simulink model "katana_smo"  (R2020a)
settings: Solver=ode8  StartTime=0.0  StopTime=20  FixedStep=0.004  MaxStep=0.004  RelTol=1e-3
InitFcn:
  | [lowpass_B, lowpass_A] = butter(4,1,'s');
  | manipulator_tree = importrobot('../../catkin_ws/src/katana_description/katana_description.urdf');
  | manipulator_tree.Gravity = [0 0 -9.81];
model workspace (MAT data in the model file):
  SL_ROS_VariableLengthArrays_MaxSizes.CommonInfo.ArrayTruncateAction = 'EmitWarning'
  SL_ROS_VariableLengthArrays_MaxSizes.MsgTypeMap = containers.Map
  SL_ROS_VariableLengthArrays_MaxSizes.MsgTypeMap.serialization.keys = {'std_msgs/Float32MultiArray', 'std_msgs/Float64MultiArray'}
  SL_ROS_VariableLengthArrays_MaxSizes.MsgTypeMap.serialization.values{1}.PropertyName = 'Data'
  SL_ROS_VariableLengthArrays_MaxSizes.MsgTypeMap.serialization.values{1}.DataType = 'single'
  SL_ROS_VariableLengthArrays_MaxSizes.MsgTypeMap.serialization.values{1}.MaxLength = 14
  SL_ROS_VariableLengthArrays_MaxSizes.MsgTypeMap.serialization.values{2}.PropertyName = 'Data'
  SL_ROS_VariableLengthArrays_MaxSizes.MsgTypeMap.serialization.values{2}.DataType = 'double'
  SL_ROS_VariableLengthArrays_MaxSizes.MsgTypeMap.serialization.values{2}.MaxLength = 7
  SL_ROS_VariableLengthArrays_MaxSizes.MsgTypeMap.serialization.uniformity = 0
  SL_ROS_VariableLengthArrays_MaxSizes.MsgTypeMap.serialization.keyType = 'char'
  SL_ROS_VariableLengthArrays_MaxSizes.MsgTypeMap.serialization.valueType = 'any'
undefined symbols (not defined in the file or in its folder): Data, Data_SL_Info, lowpass_A, lowpass_B
libraries: robotlib x9, robotmaniplib x3, robotcorelib x1
settings Model: Creator=marco  LastModifiedBy=josea
settings OptimizationCC: EnhancedBackFolding=on  PassReuseOutputArgsAs=Individual arguments  ZeroExternalMemoryAtStartup=off  ZeroInternalMemoryAtStartup=off  MaxStackSize=64  OptimizeBlockOrder=speed  DifferentSizesBufferReuse=on  OptimizationCustomize=off  EfficientTunableParamExpr=on
settings DebuggingCC: ParameterTunabilityLossMsg=error
settings HardwareCC: ProdBitPerLong=64  ProdHWDeviceType=Intel->x86-64 (Linux 64)
settings RTWCC: SystemTargetFile=ert.tlc  HardwareBoard=Robot Operating System (ROS)  TemplateMakefile=ert_default_tmf  Toolchain=Catkin  TargetLang=C++
settings CodeAppCC: ForceParamTrailComments=on  IgnoreCustomStorageClasses=off  OperatorAnnotations=on  SimulinkDataObjDesc=on  SFDataObjDesc=on  InsertBlockDesc=on
settings ERTTargetCC: SupportContinuousTime=on  SupportVariableSizeSignals=on

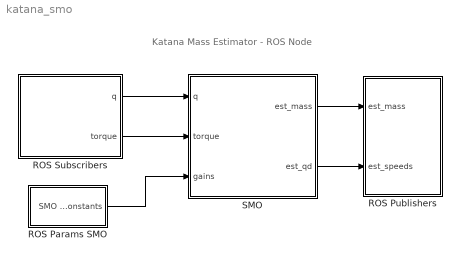
== system katana_smo ==
  note: Katana Mass Estimator - ROS Node
  ROS Params SMO : Subsystem
  ROS Publishers : Subsystem
  ROS Subscribers : Subsystem
  SMO : Subsystem
  wires:
  ROS Subscribers/2(torque) -> SMO/2(torque)
  ROS Subscribers/1(q) -> SMO/1(q)
  ROS Params SMO/1(SMO Constants) -> SMO/3(gains)
  SMO/1(est_mass) -> ROS Publishers/1(est_mass)
  SMO/2(est_qd) -> ROS Publishers/2("est_speeds ")

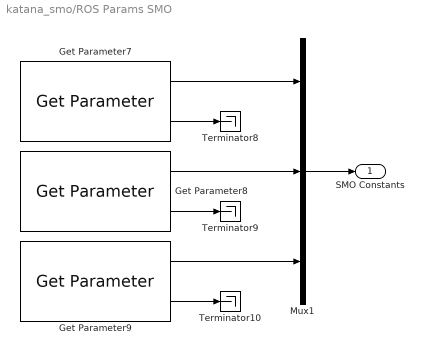
== system katana_smo/ROS Params SMO ==
  Get Parameter7 : robotlib/Get Parameter  ParameterSource=Specify your own  ParameterName=/smo/lambda  ParameterType=double  ParameterMaxArrayLength=16  ParameterInitialValue=0.0  SampleTime=1  ShowErrorCodeOutput=on  ModelName=katana_smo  BlockId=ParamGet_katana_smo_421
      settings: SourceProductBaseCode=RR
  Get Parameter8 : robotlib/Get Parameter  ParameterSource=Specify your own  ParameterName=/smo/alpha  ParameterType=double  ParameterMaxArrayLength=16  ParameterInitialValue=0.0  SampleTime=1  ShowErrorCodeOutput=on  ModelName=katana_smo  BlockId=ParamGet_katana_smo_422
      settings: SourceProductBaseCode=RR
  Get Parameter9 : robotlib/Get Parameter  ParameterSource=Specify your own  ParameterName=/smo/gamma  ParameterType=double  ParameterMaxArrayLength=16  ParameterInitialValue=0.0  SampleTime=1  ShowErrorCodeOutput=on  ModelName=katana_smo  BlockId=ParamGet_katana_smo_423
      settings: SourceProductBaseCode=RR
  Mux1 : Mux  Inputs=3
  Terminator10 : Terminator
  Terminator8 : Terminator
  Terminator9 : Terminator
  SMO Constants : Outport
  wires:
  Get Parameter9/1 -> Mux1/3
  Get Parameter7/1 -> Mux1/1
  Get Parameter7/2 -> Terminator8/1
  Mux1/1 -> SMO Constants/1
  Get Parameter8/2 -> Terminator9/1
  Get Parameter9/2 -> Terminator10/1
  Get Parameter8/1 -> Mux1/2

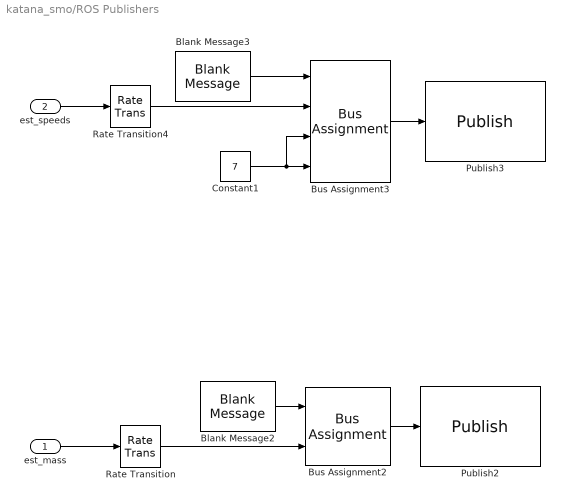
== system katana_smo/ROS Publishers ==
  est_mass : Inport
  "est_speeds " : Inport  Port=2
  Blank Message2 : robotlib/Blank Message  messageClass=Message  entityType=std_msgs/Float64  messageType=std_msgs/Float64  SampleTime=0.04
  Blank Message3 : robotlib/Blank Message  messageClass=Message  entityType=std_msgs/Float64MultiArray  messageType=std_msgs/Float64MultiArray  SampleTime=0.004
  Bus Assignment2 : BusAssignment  AssignedSignals=Data
  Bus Assignment3 : BusAssignment  AssignedSignals=Data,Data_SL_Info.CurrentLength,Data_SL_Info.ReceivedLength
  Constant1 : Constant  Value=7  OutDataTypeStr=uint32  SampleTime=0.004
  Publish2 : robotlib/Publish  topicSource=Specify your own  topic=/estimated_mass  messageType=std_msgs/Float64  messageQueueLength=1
  Publish3 : robotlib/Publish  topicSource=Specify your own  topic=/smo/estimated_speeds  messageType=std_msgs/Float64MultiArray  messageQueueLength=1
  Rate Transition : RateTransition
  Rate Transition4 : RateTransition
  wires:
  Blank Message2/1 -> Bus Assignment2/1
  Rate Transition/1 -> Bus Assignment2/2
  Bus Assignment2/1 -> Publish2/1
  Rate Transition4/1 -> Bus Assignment3/2
  Bus Assignment3/1 -> Publish3/1
  Constant1/1 -> Bus Assignment3/4, Bus Assignment3/3
  Blank Message3/1 -> Bus Assignment3/1
  est_mass/1 -> Rate Transition/1
  "est_speeds "/1 -> Rate Transition4/1

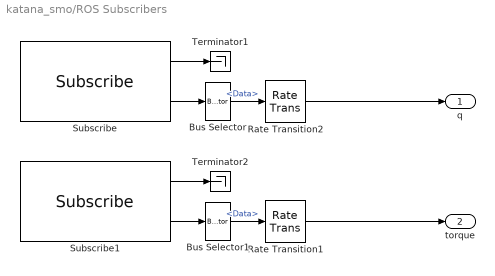
== system katana_smo/ROS Subscribers ==
  Bus Selector : BusSelector  OutputSignals=Data
  Bus Selector1 : BusSelector  OutputSignals=Data
  Rate Transition1 : RateTransition
  Rate Transition2 : RateTransition
  Subscribe : robotlib/Subscribe  topicSource=Specify your own  topic=/joint_positions  messageType=std_msgs/Float64MultiArray  sampleTime=0.004  messageQueueLength=1
  Subscribe1 : robotlib/Subscribe  topicSource=Specify your own  topic=/joint_torques  messageType=std_msgs/Float64MultiArray  sampleTime=0.004  messageQueueLength=1
  Terminator1 : Terminator
  Terminator2 : Terminator
  q : Outport
  torque : Outport  Port=2
  wires:
  Bus Selector/1 -> Rate Transition2/1  "<Data>"
  Rate Transition2/1 -> q/1
  Subscribe/2 -> Bus Selector/1
  Subscribe/1 -> Terminator1/1
  Subscribe1/1 -> Terminator2/1
  Subscribe1/2 -> Bus Selector1/1
  Bus Selector1/1 -> Rate Transition1/1  "<Data>"
  Rate Transition1/1 -> torque/1

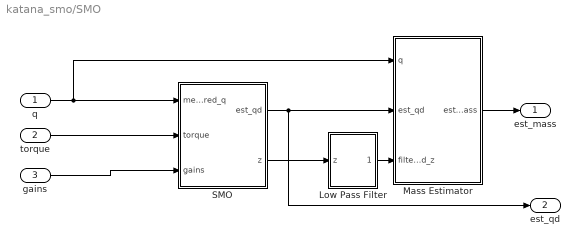
== system katana_smo/SMO ==
  q : Inport
  torque : Inport  Port=2
  gains : Inport  Port=3
  Low Pass Filter : Subsystem
  Mass Estimator : Subsystem
  SMO : Subsystem
  est_mass : Outport
  est_qd : Outport  Port=2
  wires:
  SMO/2(z) -> Low Pass Filter/1(z)
  Mass Estimator/1(est_mass) -> est_mass/1
  torque/1 -> SMO/2(torque)
  q/1 -> Mass Estimator/1(q), SMO/1(measured_q)
  Low Pass Filter/1(filtered) -> Mass Estimator/3(filtered_z)
  gains/1 -> SMO/3(gains)
  SMO/1(est_qd) -> est_qd/1, Mass Estimator/2(est_qd)

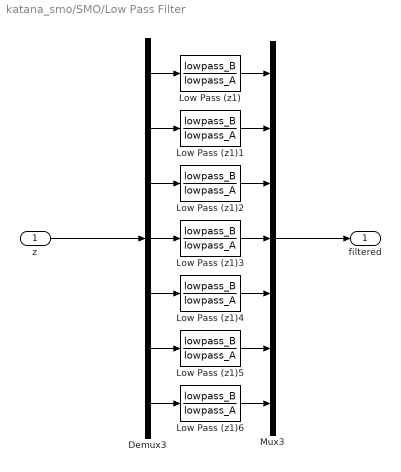
== system katana_smo/SMO/Low Pass Filter ==
  z : Inport
  Demux3 : Demux  Outputs=7
  Low Pass (z1){,1..6} (7 alike) : TransferFcn  Numerator=lowpass_B  Denominator=lowpass_A
  Mux3 : Mux  Inputs=7
  filtered : Outport
  wires:
  Demux3/1 -> Low Pass (z1)/1
  Low Pass (z1)5/1 -> Mux3/6
  Low Pass (z1)2/1 -> Mux3/3
  Demux3/6 -> Low Pass (z1)5/1
  Low Pass (z1)4/1 -> Mux3/5
  z/1 -> Demux3/1
  Demux3/7 -> Low Pass (z1)6/1
  Demux3/5 -> Low Pass (z1)4/1
  Low Pass (z1)/1 -> Mux3/1
  Demux3/2 -> Low Pass (z1)1/1
  Mux3/1 -> filtered/1
  Low Pass (z1)6/1 -> Mux3/7
  Low Pass (z1)1/1 -> Mux3/2
  Demux3/4 -> Low Pass (z1)3/1
  Low Pass (z1)3/1 -> Mux3/4
  Demux3/3 -> Low Pass (z1)2/1

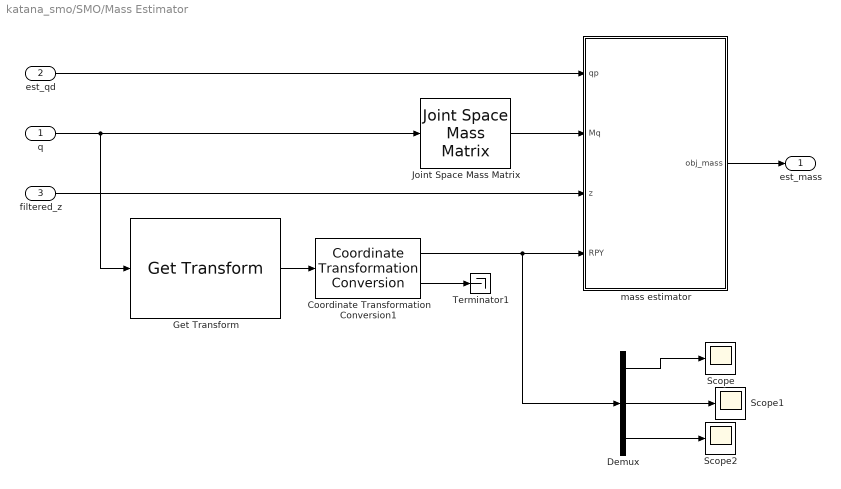
== system katana_smo/SMO/Mass Estimator ==
  q : Inport
  est_qd : Inport  Port=2
  filtered_z : Inport  Port=3
  Coordinate Transformation Conversion1 : robotcorelib/Coordinate Transformation Conversion  InputRepresentation=Homogeneous Transformation  InputEulerSequence=ZYX  ShowTrVecInputPort=on  OutputRepresentation=Euler Angles  OutputEulerSequence=ZYX  ShowTrVecOutputPort=on  SimulateUsing=Code generation
      settings: SourceProductBaseCode=NV,RO,RR
  Demux : Demux  Outputs=3
  Get Transform : robotmaniplib/Get Transform  RigidBodyTree=manipulator_tree  SourceBody=katana_base_frame  TargetBody=katana_motor4_lift_link  SimulateUsing=Code generation
  Joint Space Mass Matrix : robotmaniplib/Joint Space Mass Matrix  RigidBodyTree=manipulator_tree  SimulateUsing=Code generation
  Scope : Scope
  Scope1 : Scope
  Scope2 : Scope
  Terminator1 : Terminator
  mass estimator : MATLAB Function  TreatAsAtomicUnit=on
  est_mass : Outport
  wires:
  Get Transform/1 -> Coordinate Transformation Conversion1/1
  Joint Space Mass Matrix/1 -> mass estimator/2(Mq)
  q/1 -> Get Transform/1, Joint Space Mass Matrix/1
  mass estimator/1(obj_mass) -> est_mass/1
  est_qd/1 -> mass estimator/1(qp)
  filtered_z/1 -> mass estimator/3(z)
  Coordinate Transformation Conversion1/2 -> Terminator1/1
  Coordinate Transformation Conversion1/1 -> Demux/1, mass estimator/4(RPY)
  Demux/3 -> Scope2/1
  Demux/2 -> Scope1/1
  Demux/1 -> Scope/1

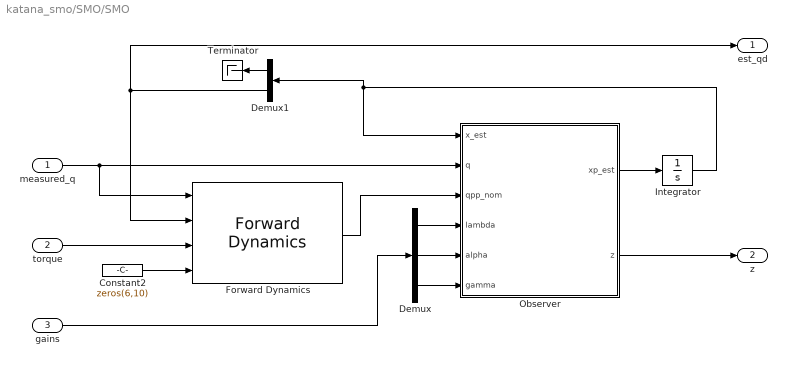
== system katana_smo/SMO/SMO ==
  measured_q : Inport
  torque : Inport  Port=2
  gains : Inport  Port=3
  Constant2 : Constant  Value=zeros(6,10)  SampleTime=-1
  Demux : Demux  Outputs=3
  Demux1 : Demux  Outputs=[7,7]
  Forward Dynamics : robotmaniplib/Forward Dynamics  RigidBodyTree=manipulator_tree  SimulateUsing=Code generation
  Integrator : Integrator  InitialCondition=[0 0 0 0 0 0 0 0 0 0 0 0 0 0]
  Observer : MATLAB Function  TreatAsAtomicUnit=on
  Terminator : Terminator
  est_qd : Outport
  z : Outport  Port=2
  wires:
  gains/1 -> Demux/1
  Demux/1 -> Observer/4(lambda)
  Demux/2 -> Observer/5(alpha)
  Demux/3 -> Observer/6(gamma)
  Demux1/2 -> Forward Dynamics/2, est_qd/1
  measured_q/1 -> Observer/2(q), Forward Dynamics/1
  Observer/2(z) -> z/1
  torque/1 -> Forward Dynamics/3
  Integrator/1 -> Observer/1(x_est), Demux1/1
  Forward Dynamics/1 -> Observer/3(qpp_nom)
  Observer/1(xp_est) -> Integrator/1
  Demux1/1 -> Terminator/1
  Constant2/1 -> Forward Dynamics/4

== matlab function katana_smo/SMO/SMO/Observer ==
  data: x_est input; q input; qpp_nom input; xp_est output; z output; lambda input; alpha input; gamma input
function [xp_est, z] = observer(x_est, q, qpp_nom, lambda, alpha, gamma)
xp_est = zeros(14,1);
q_est  = x_est(1:7);
qp_est = x_est(8:14);
z1 = zeros(1,7);
z2 = zeros(1,7);

%lambda = 10;
%alpha  = 10;
%lambda = 6;
%alpha  = 4.2;
%gamma = 0.001;

for i=1:7
    %z1(i) = lambda*sqrt(abs(q(i) - q_est(i)))*sign(q(i) - q_est(i));
    %z2(i) = alpha*sign(q(i) - q_est(i));
    z1(i) = lambda*sqrt(abs(q(i) - q_est(i)))*(2/(1 + exp((q_est(i) - q(i))/gamma)) - 1);
    z2(i) = alpha*(2/(1 + exp((q_est(i) - q(i))/gamma)) - 1);
end

for i=1:7
    xp_est(i)   = qp_est(i) + z1(i);
    xp_est(i+7) = qpp_nom(i) + z2(i);
end

z = z2;

== matlab function katana_smo/SMO/Mass Estimator/mass estimator ==
  data: qp input; Mq input; z input; RPY input; obj_mass output
function obj_mass = mass_est(qp, Mq, z, RPY)
phi = Mq*z;
g = 9.81;
l = 0.2596; % = distance from joint 4 to joint 5, plus joint 5 to gripper, plus gripper joint to gripper center. (Check in urdf)
pitch = RPY(1);

if abs(cos(pitch)) > 0.2
    obj_mass = phi(4)/(l*g*cos(pitch));
else
    obj_mass = 0;
end
